simulink model "karina"  (R2022a)
settings: Solver=FixedStepAuto  StartTime=0.0  StopTime=500  FixedStep=0.001  RelTol=1e-3
libraries: slpidlib x1
settings Model: Creator=Userx  LastModifiedBy=Userx

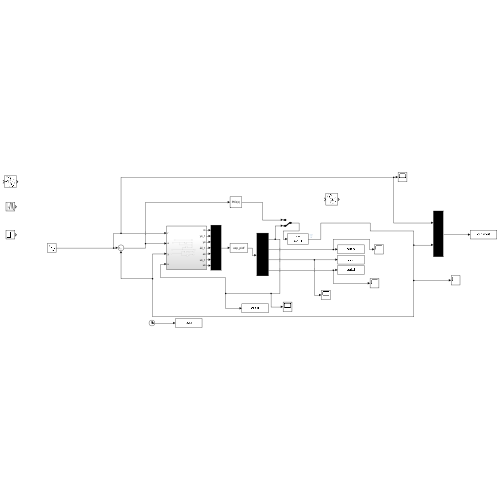
[thumbnail: Simulink's stored preview of the top-level diagram]
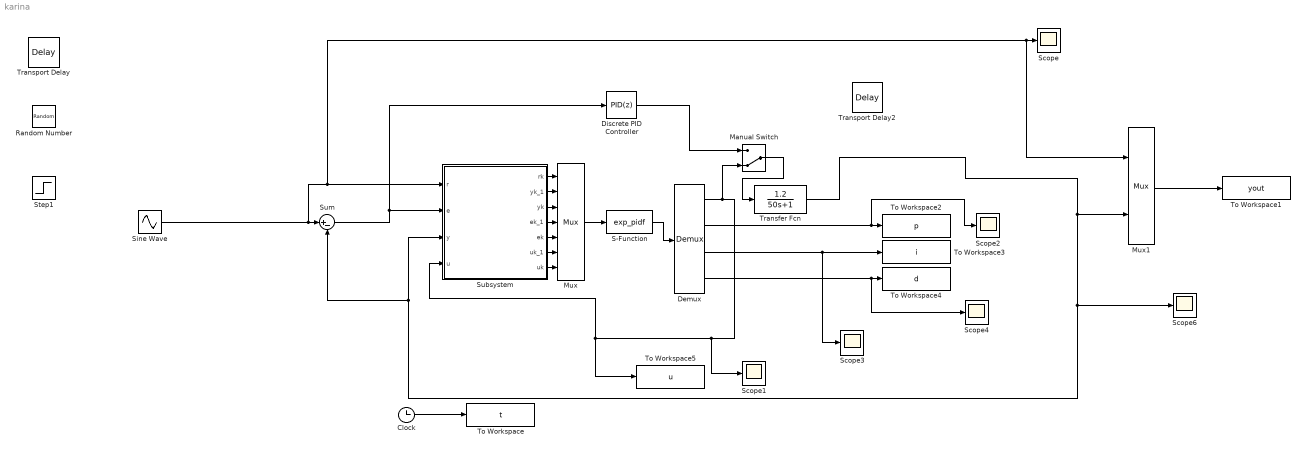
== system karina ==
  Clock : Clock
  Demux : Demux
  Discrete PID Controller : slpidlib/PID Controller  Controller=PID  Form=Parallel  TimeDomain=Discrete-time  UseExternalTs=off  SampleTime=-1  IntegratorMethod=Forward Euler  FilterMethod=Forward Euler  ControllerParametersSource=internal  P=10  I=5  UseKiTs=off  D=2  N=100  UseFilter=off  TunerSelectOption=Transfer Function Based (PID Tuner App)  InitialConditionSource=internal  InitialConditionForIntegrator=0  InitialConditionForFilter=0  DifferentiatorICPrevScaledInput=0  ExternalReset=none  TrackingMode=off  Kt=1  LimitOutput=off  SatLimitsSource=internal  UpperSaturationLimit=inf  LowerSaturationLimit=-inf  LinearizeAsGain=off  AntiWindupMode=none  Kb=1  POutMin=[]  POutMax=[]  IOutMin=[]  IOutMax=[]  DOutMin=[]  DOutMax=[]  NOutMin=[]  NOutMax=[]  SumOutMin=[]  SumOutMax=[]  SaturationOutMin=[]  SaturationOutMax=[]  PParamMin=[]  PParamMax=[]  IParamMin=[]  IParamMax=[]  DParamMin=[]  DParamMax=[]  NParamMin=[]  NParamMax=[]  KbParamMin=[]  KbParamMax=[]  KtParamMin=[]  KtParamMax=[]  KbOutMin=[]  KbOutMax=[]  KtOutMin=[]  KtOutMax=[]  IntegratorOutMin=[]  IntegratorOutMax=[]  FilterOutMin=[]  FilterOutMax=[]  SumI1OutMin=[]  SumI1OutMax=[]  SumI2OutMin=[]  SumI2OutMax=[]  SumI3OutMin=[]  SumI3OutMax=[]  SumI4OutMin=[]  SumI4OutMax=[]  SumDOutMin=[]  SumDOutMax=[]  DifferentiatorOutMin=[]  DifferentiatorOutMax=[]  FilterDiffOutCoefMin=[]  FilterDiffOutCoefMax=[]  ReciprocalOutMin=[]  ReciprocalOutMax=[]  SumDenOutMin=[]  SumDenOutMax=[]  SumNumOutMin=[]  SumNumOutMax=[]  DivideOutMin=[]  DivideOutMax=[]  UdiffTsProdOutMin=[]  UdiffTsProdOutMax=[]  NTsProdOutMin=[]  NTsProdOutMax=[]  UintegralTsProdOutMin=[]  UintegralTsProdOutMax=[]  UngainTsProdOutMin=[]  UngainTsProdOutMax=[]  IntegratorContinuousStateAttributes=''  IntegratorStateMustResolveToSignalObject=off  IntegratorRTWStateStorageClass=Auto  FilterContinuousStateAttributes=''  FilterStateMustResolveToSignalObject=off  FilterRTWStateStorageClass=Auto  ParallelPVariant=InternalParameters  IdealPVariant=Disabled  IVariant=InternalParameters  DVariant=InternalParameters  IntegratorVariant=Discrete  SatVariant=Disabled  AWVariant=Passthrough  PCopyVariant=Disabled  TRVariant=Disabled  FdbkBlocksVariant=Forward  IdealPFdbkVariant=Disabled  SatFdbkVariant=Disabled  DerivativeFilterVariant=Differentiator  NVariant=Passthrough  NCopyVariant=Disabled_SignalSpec  FilterICVariant=InternalICsDifferentiator  IntegratorICVariant=InternalICs  ExternalResetVariant=Disabled  TRSumVariant=Passthrough  SumFdbkVariant=Disabled  SumVariant=Sum_PID  TsampFilterVariant=InternalTs  TsampNgainVariant=Passthrough  TsampIntegralVariant=Passthrough  ExternalSaturationOutDataTypeStr=Inherit: Same as second input  aMode=0
  Manual Switch : ManualSwitch  CurrentSetting=0
  Mux : Mux  Inputs=7
  Mux1 : Mux  Inputs=2
  Random Number : RandomNumber  Variance=0.01  SampleTime=0.1
  S-Function : S-Function  FunctionName=exp_pidf  SFunctionDeploymentMode=off  EnableBusSupport=off
  Scope{,1..4,6} (6 alike) : Scope
  Sine Wave : Sin  Frequency=0.02  SampleTime=0
  Step1 : Step  SampleTime=0
  Subsystem : Subsystem
  Sum : Sum  Inputs=|+-
  To Workspace : ToWorkspace  VariableName=t  SampleTime=-1
  To Workspace1 : ToWorkspace  VariableName=yout  SaveFormat=Timeseries  SampleTime=-1
  To Workspace2 : ToWorkspace  VariableName=p  SampleTime=-1
  To Workspace3 : ToWorkspace  VariableName=i  SampleTime=-1
  To Workspace4 : ToWorkspace  VariableName=d  SampleTime=-1
  To Workspace5 : ToWorkspace  VariableName=u  SampleTime=-1
  Transfer Fcn : TransferFcn  Numerator=[1.2]  Denominator=[50 1]
  Transport Delay : TransportDelay
  Transport Delay2 : TransportDelay  DelayTime=20
  wires:
  Mux/1 -> S-Function/1
  S-Function/1 -> Demux/1
  Demux/1 -> Manual Switch/2, Scope1/1, Subsystem/4(u), To Workspace5/1
  Mux1/1 -> To Workspace1/1
  Demux/2 -> Scope2/1, To Workspace2/1
  Demux/3 -> To Workspace3/1, Scope3/1
  Demux/4 -> Scope4/1, To Workspace4/1
  Subsystem/1(rk) -> Mux/1
  Subsystem/2(yk_1) -> Mux/2
  Subsystem/3(yk) -> Mux/3
  Subsystem/4(ek_1) -> Mux/4
  Subsystem/5(ek) -> Mux/5
  Subsystem/6(uk_1) -> Mux/6
  Subsystem/7(uk) -> Mux/7
  Sum/1 -> Subsystem/2(e), Discrete PID Controller/1
  Clock/1 -> To Workspace/1
  Sine Wave/1 -> Mux1/1, Scope/1, Subsystem/1(r), Sum/1
  Discrete PID Controller/1 -> Manual Switch/1
  Manual Switch/1 -> Transfer Fcn/1
  Transfer Fcn/1 -> Subsystem/3(y), Sum/2, Scope6/1, Mux1/2

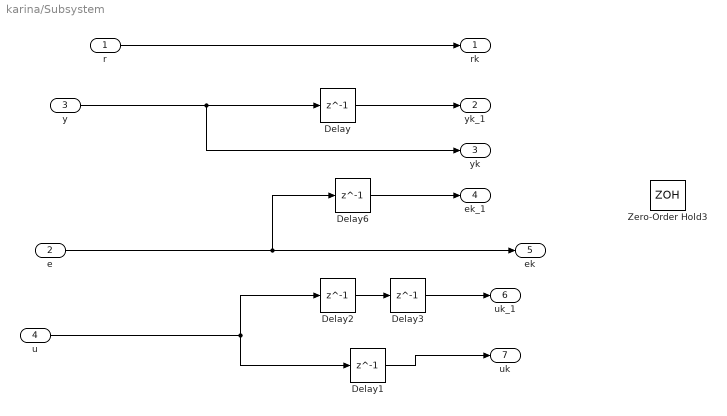
== system karina/Subsystem ==
  r : Inport
  e : Inport  Port=2
  y : Inport  Port=3
  u : Inport  Port=4
  Delay{,1..3,6} (5 alike) : Delay  DelayLength=1
  Zero-Order Hold3 : ZeroOrderHold  SampleTime=-1
  rk : Outport
  yk_1 : Outport  Port=2
  yk : Outport  Port=3
  ek_1 : Outport  Port=4
  ek : Outport  Port=5
  uk_1 : Outport  Port=6
  uk : Outport  Port=7
  wires:
  u/1 -> Delay1/1, Delay2/1
  Delay6/1 -> ek_1/1
  Delay/1 -> yk_1/1
  r/1 -> rk/1
  e/1 -> ek/1, Delay6/1
  y/1 -> yk/1, Delay/1
  Delay3/1 -> uk_1/1
  Delay1/1 -> uk/1
  Delay2/1 -> Delay3/1
